simulink model "LICENTA_2024v8"  (R2018b)
settings: Solver=FixedStepDiscrete  StartTime=0.0  StopTime=Inf  RelTol=1e-3  EnableMultiTasking=on
values from neighbouring files (symbols this model uses):
  factor_conversie = (1/Rshunt)*(1/10)*(vref/4095)    (= 0.0115122972266)    [licentam18.m]
  FED = uint16(50)    [licentam18.m]
  MaxIter_1_ms_eCAP_wait = MinDetectSpeed_period/T_pos    (= 375)    [licentam18.m]
  offset_ADC = xT*4095/vref    (= 2047.5)    [licentam18.m]
  pp = 16/2    (= 8)    [licentam18.m]
  RED = uint16(50)    [licentam18.m]
  T_pos = 5*10^-4    (= 0.0005)    [licentam18.m]
  TBPRD1 = uint16(TPWM/(2*TTBCLK))    [licentam18.m]
  Tf = 0.015    [licentam18.m]
  Tf_spd = 0.01    [licentam18.m]
  TiSamplePos = T_pos    (= 0.0005)    [licentam18.m]
  Ts = Ts_crt_control    (= 3.33333333333e-05)    [licentam18.m]
  TTBCLK = 1/F    (= 5e-09)    [licentam18.m]
undefined symbols (not defined in the file or in its folder): Discrete, Down, GPTRIP1SEL, GPTRIP2SEL, radians, Time, TZ1, TZ2, Up
libraries: tiiqmathlib x25, c2802xlib x6, c2837xDlib x6, c280xlib x4, simulink x3, ctrlSharedLib x2, c2000lib x1, c28xdmclib x1
(part 2 of 2)

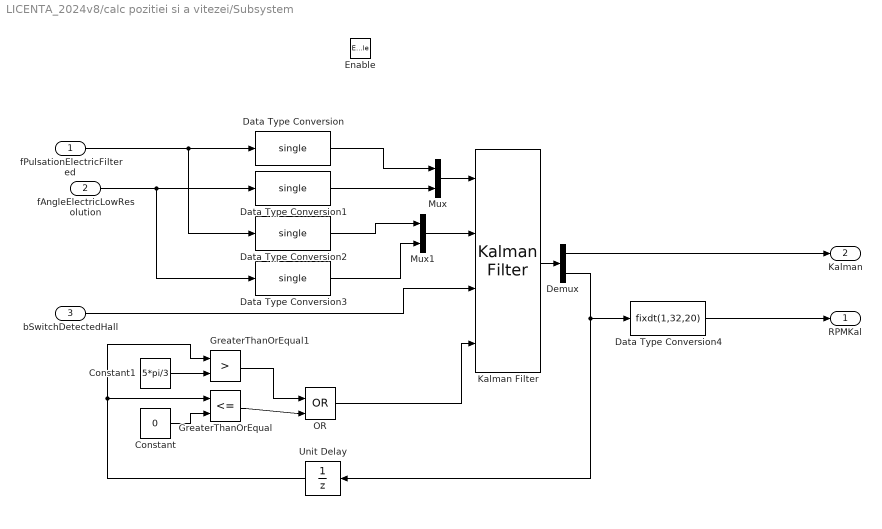
== system LICENTA_2024v8/calc pozitiei si a vitezei/Subsystem ==
  fPulsationElectricFiltered : Inport
  fAngleElectricLowResolution : Inport  Port=2
  bSwitchDetectedHall : Inport  Port=3
  Enable : EnablePort  StatesWhenEnabling=reset
  Constant : Constant  Value=0
  Constant1 : Constant  Value=5*pi/3
  Data Type Conversion{,1..3} (4 alike) : DataTypeConversion  OutDataTypeStr=single
  Data Type Conversion4 : DataTypeConversion  OutDataTypeStr=fixdt(1,32,20)
  Demux : Demux  Outputs=2
  GreaterThanOrEqual : RelationalOperator  Operator=<=  OutDataTypeStr=boolean  RndMeth=Simplest
  GreaterThanOrEqual1 : RelationalOperator  Operator=>  OutDataTypeStr=boolean  RndMeth=Simplest
  Kalman Filter : ctrlSharedLib/Kalman Filter  TimeDomain=Discrete-Time  UseCurrentEstimator=on  ModelSource=Individual A, B, C, D matrices  ModelSourceVariable=ss(0.95,1,1,0,1)  A=[1, 0; TiSamplePos 1]  B=1  C=eye(2)  D=0  NumberOfStates=1  NumberOfInputs=1  NumberOfOutputs=1  InitialEstimateSource=Input port  X0=0  P0=10  UseK=off  UseGH=off  NumberOfProcessNoiseInputs=1  G=1  TimeInvariantG=on  H=0  TimeInvariantH=on  Q=diag([0.00005 0.02])  TimeInvariantQ=on  R=diag([0.02 0.002])  TimeInvariantR=on  N=0  TimeInvariantN=on  AddInputPort=off  AddEnablePort=on  ExternalReset=Rising  OutputEstimatedY=off  OutputP=off  Ts=-1
      settings: SourceProductBaseCode=CT
  Mux : Mux  Inputs=2
  Mux1 : Mux  Inputs=2
  OR : Logic  Operator=OR  IconShape=distinctive  AllPortsSameDT=off  OutDataTypeStr=boolean
  Unit Delay : UnitDelay  SampleTime=-1
  RPMKal : Outport  VectorParamsAs1DForOutWhenUnconnected=on
  Kalman : Outport  Port=2
  wires:
  Kalman Filter/1 -> Demux/1
  Data Type Conversion3/1 -> Mux1/2
  Unit Delay/1 -> GreaterThanOrEqual/1, GreaterThanOrEqual1/1
  Data Type Conversion/1 -> Mux/1
  Constant/1 -> GreaterThanOrEqual/2
  Data Type Conversion1/1 -> Mux/2
  Data Type Conversion2/1 -> Mux1/1
  GreaterThanOrEqual/1 -> OR/2
  Constant1/1 -> GreaterThanOrEqual1/2
  Data Type Conversion4/1 -> RPMKal/1
  Mux/1 -> Kalman Filter/1
  Mux1/1 -> Kalman Filter/2
  OR/1 -> Kalman Filter/4
  GreaterThanOrEqual1/1 -> OR/1
  Demux/1 -> Kalman/1
  Demux/2 -> Unit Delay/1, Data Type Conversion4/1
  bSwitchDetectedHall/1 -> Kalman Filter/3
  fPulsationElectricFiltered/1 -> Data Type Conversion2/1, Data Type Conversion/1
  fAngleElectricLowResolution/1 -> Data Type Conversion3/1, Data Type Conversion1/1

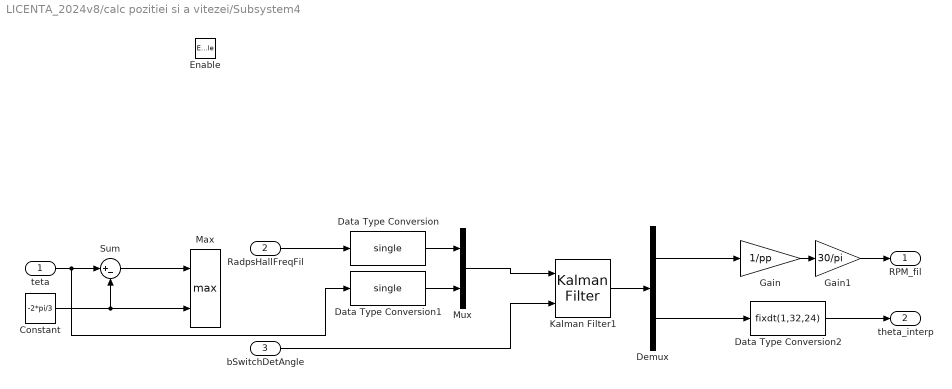
== system LICENTA_2024v8/calc pozitiei si a vitezei/Subsystem4 ==
  "teta " : Inport
  RadpsHallFreqFil : Inport  Port=2
  bSwitchDetAngle : Inport  Port=3
  Enable : EnablePort
  Constant : Constant  Value=-2*pi/3
  Data Type Conversion : DataTypeConversion  OutDataTypeStr=single
  Data Type Conversion1 : DataTypeConversion  OutDataTypeStr=single
  Data Type Conversion2 : DataTypeConversion  OutDataTypeStr=fixdt(1,32,24)
  Demux : Demux  Outputs=2
  Gain : Gain  Gain=1/pp
  Gain1 : Gain  Gain=30/pi
  Kalman Filter1 : ctrlSharedLib/Kalman Filter  TimeDomain=Discrete-Time  UseCurrentEstimator=on  ModelSource=Individual A, B, C, D matrices  ModelSourceVariable=sys  A=[1, 0; TiSamplePos 1]  B=eye(2)  C=eye(2)  D=zeros(2)  NumberOfStates=2  NumberOfInputs=2  NumberOfOutputs=2  InitialEstimateSource=Dialog  X0=0  P0=10  UseK=off  UseGH=off  NumberOfProcessNoiseInputs=2  G=1  TimeInvariantG=on  H=0  TimeInvariantH=on  Q=diag([0.2 0.5])  TimeInvariantQ=on  R=diag([2.5 0.001])  TimeInvariantR=on  N=0  TimeInvariantN=on  AddInputPort=off  AddEnablePort=on  OutputEstimatedY=off  OutputP=off  Ts=-1
      settings: SourceProductBaseCode=CT
  Max : MinMax  Function=max  Inputs=2
  Mux : Mux  Inputs=2
  Sum : Sum  Inputs=|+-
  RPM_fil : Outport
  theta_interp : Outport  Port=2
  wires:
  Data Type Conversion2/1 -> theta_interp/1
  Gain1/1 -> RPM_fil/1
  Demux/2 -> Data Type Conversion2/1
  Gain/1 -> Gain1/1
  Demux/1 -> Gain/1
  Kalman Filter1/1 -> Demux/1
  bSwitchDetAngle/1 -> Kalman Filter1/2
  Mux/1 -> Kalman Filter1/1
  Data Type Conversion1/1 -> Mux/2
  Data Type Conversion/1 -> Mux/1
  RadpsHallFreqFil/1 -> Data Type Conversion/1
  Sum/1 -> Max/1
  Constant/1 -> Max/2, Sum/2
  "teta "/1 -> Data Type Conversion1/1, Sum/1

== system LICENTA_2024v8/calc pozitiei si a vitezei/calc pozitie ==
  In1 : Inport
  Data Type Conversion : DataTypeConversion  OutDataTypeStr=int8
  MATLAB Function : MATLAB Function  TreatAsAtomicUnit=on
  citire senzori hall & calcul teta : Subsystem
  gradient : Subsystem
  teta : Outport  VectorParamsAs1DForOutWhenUnconnected=on
  int8dir : Outport  Port=2  VectorParamsAs1DForOutWhenUnconnected=on
  "seq. change detected " : Outport  Port=3  VectorParamsAs1DForOutWhenUnconnected=on
  wires:
  Data Type Conversion/1 -> int8dir/1
  MATLAB Function/1(dir) -> Data Type Conversion/1
  gradient/1(gradient) -> MATLAB Function/1(u)
  citire senzori hall & calcul teta/1(teta) -> teta/1, gradient/1(teta)
  citire senzori hall & calcul teta/2("seq. change detected ") -> "seq. change detected "/1, gradient/Trigger
  In1/1 -> citire senzori hall & calcul teta/1(In1)

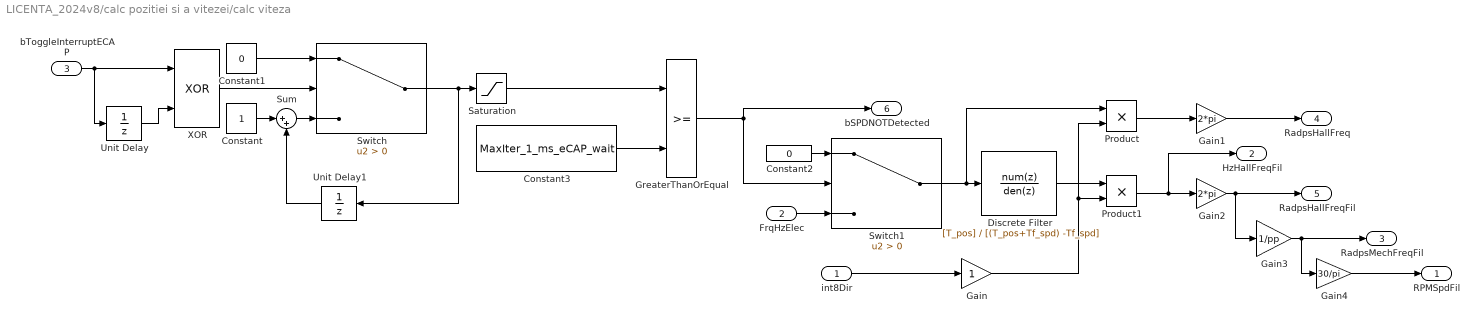
== system LICENTA_2024v8/calc pozitiei si a vitezei/calc viteza ==
  int8Dir : Inport
  FrqHzElec : Inport  Port=2
  bToggleInterruptECAP : Inport  Port=3
  Constant : Constant
  Constant1 : Constant  Value=0
  Constant2 : Constant  Value=0
  Constant3 : Constant  Value=MaxIter_1_ms_eCAP_wait
  Discrete Filter : DiscreteFilter  Numerator=[T_pos]  Denominator=[(T_pos+Tf_spd) -Tf_spd]
  Gain : Gain
  Gain1 : Gain  Gain=2*pi
  Gain2 : Gain  Gain=2*pi
  Gain3 : Gain  Gain=1/pp
  Gain4 : Gain  Gain=30/pi
  GreaterThanOrEqual : RelationalOperator  OutDataTypeStr=boolean  RndMeth=Simplest
  Product : Product
  Product1 : Product
  Saturation : Saturate  UpperLimit=MaxIter_1_ms_eCAP_wait  LowerLimit=0
  Sum : Sum  Inputs=|++
  Switch : Switch  Criteria=u2 > Threshold
  Switch1 : Switch  Criteria=u2 > Threshold
  Unit Delay : UnitDelay  SampleTime=-1
  Unit Delay1 : UnitDelay  SampleTime=-1
  XOR : Logic  Operator=XOR  IconShape=distinctive  AllPortsSameDT=off  OutDataTypeStr=boolean
  RPMSpdFil : Outport  VectorParamsAs1DForOutWhenUnconnected=on
  HzHallFreqFil : Outport  Port=2  VectorParamsAs1DForOutWhenUnconnected=on
  RadpsMechFreqFil : Outport  Port=3  VectorParamsAs1DForOutWhenUnconnected=on
  RadpsHallFreq : Outport  Port=4  VectorParamsAs1DForOutWhenUnconnected=on
  RadpsHallFreqFil : Outport  Port=5  VectorParamsAs1DForOutWhenUnconnected=on
  bSPDNOTDetected : Outport  Port=6  VectorParamsAs1DForOutWhenUnconnected=on
  wires:
  Constant2/1 -> Switch1/1
  FrqHzElec/1 -> Switch1/3
  Sum/1 -> Switch/3
  Unit Delay/1 -> XOR/2
  Saturation/1 -> GreaterThanOrEqual/1
  bToggleInterruptECAP/1 -> XOR/1, Unit Delay/1
  Unit Delay1/1 -> Sum/2
  Switch/1 -> Unit Delay1/1, Saturation/1
  Constant/1 -> Sum/1
  Product1/1 -> Gain2/1, HzHallFreqFil/1
  XOR/1 -> Switch/2
  Product/1 -> Gain1/1
  Constant3/1 -> GreaterThanOrEqual/2
  Gain1/1 -> RadpsHallFreq/1
  Gain/1 -> Product1/2, Product/2
  Constant1/1 -> Switch/1
  Gain4/1 -> RPMSpdFil/1
  Gain2/1 -> Gain3/1, RadpsHallFreqFil/1
  GreaterThanOrEqual/1 -> Switch1/2, bSPDNOTDetected/1
  Gain3/1 -> Gain4/1, RadpsMechFreqFil/1
  Discrete Filter/1 -> Product1/1
  int8Dir/1 -> Gain/1
  Switch1/1 -> Product/1, Discrete Filter/1

== system LICENTA_2024v8/eCAP/If Action Subsystem ==
  HzHallFreqPrev : Inport
  Action Port : ActionPort  ActionType=then
  HzHallFreq : Outport  VectorParamsAs1DForOutWhenUnconnected=on
  wires:
  HzHallFreqPrev/1 -> HzHallFreq/1

== system LICENTA_2024v8/eCAP/If Action Subsystem1 ==
  Action Port : ActionPort  ActionType=elseif
  Constant : Constant  Value=0
  HzHallFreq : Outport  VectorParamsAs1DForOutWhenUnconnected=on
  wires:
  Constant/1 -> HzHallFreq/1

== system LICENTA_2024v8/eCAP/If Action Subsystem2 ==
  HallPeriod : Inport
  Action Port : ActionPort  ActionType=else
  Constant : Constant
  Multiply : Product  Inputs=*/
  HzHallFreq : Outport  VectorParamsAs1DForOutWhenUnconnected=on
  wires:
  HallPeriod/1 -> Multiply/2
  Constant/1 -> Multiply/1
  Multiply/1 -> HzHallFreq/1

== system LICENTA_2024v8/calc pozitiei si a vitezei/calc pozitie/citire senzori hall & calcul teta ==
  In1 : Inport
  Digital Input : c2837xDlib/Digital Input  GPIO_Number=GPIO24~GPIO31  GPIO_Bit0=off  GPIO_Bit1=off  GPIO_Bit2=on  GPIO_Bit3=off  GPIO_Bit4=off  GPIO_Bit5=off  GPIO_Bit6=off  GPIO_Bit7=off  sampleTime=-1  dataType=auto  GPIO_Bit0_Qualification=Sync to SYSCLKOUT  GPIO_Bit1_Qualification=Sync to SYSCLKOUT  GPIO_Bit2_Qualification=Sync to SYSCLKOUT  GPIO_Bit3_Qualification=Sync to SYSCLKOUT  GPIO_Bit4_Qualification=Sync to SYSCLKOUT  GPIO_Bit5_Qualification=Sync to SYSCLKOUT  GPIO_Bit6_Qualification=Sync to SYSCLKOUT  GPIO_Bit7_Qualification=Sync to SYSCLKOUT  Qualification_Period=-1
      settings: SourceProductBaseCode=TIC2000
  Digital Input1 : c2837xDlib/Digital Input  GPIO_Number=GPIO24~GPIO31  GPIO_Bit0=off  GPIO_Bit1=off  GPIO_Bit2=off  GPIO_Bit3=on  GPIO_Bit4=off  GPIO_Bit5=off  GPIO_Bit6=off  GPIO_Bit7=off  sampleTime=-1  dataType=auto  GPIO_Bit0_Qualification=Sync to SYSCLKOUT  GPIO_Bit1_Qualification=Sync to SYSCLKOUT  GPIO_Bit2_Qualification=Sync to SYSCLKOUT  GPIO_Bit3_Qualification=Sync to SYSCLKOUT  GPIO_Bit4_Qualification=Sync to SYSCLKOUT  GPIO_Bit5_Qualification=Sync to SYSCLKOUT  GPIO_Bit6_Qualification=Sync to SYSCLKOUT  GPIO_Bit7_Qualification=Sync to SYSCLKOUT  Qualification_Period=-1
      settings: SourceProductBaseCode=TIC2000
  Digital Input2 : c2837xDlib/Digital Input  GPIO_Number=GPIO24~GPIO31  GPIO_Bit0=off  GPIO_Bit1=on  GPIO_Bit2=off  GPIO_Bit3=off  GPIO_Bit4=off  GPIO_Bit5=off  GPIO_Bit6=off  GPIO_Bit7=off  sampleTime=-1  dataType=auto  GPIO_Bit0_Qualification=Sync to SYSCLKOUT  GPIO_Bit1_Qualification=Sync to SYSCLKOUT  GPIO_Bit2_Qualification=Sync to SYSCLKOUT  GPIO_Bit3_Qualification=Sync to SYSCLKOUT  GPIO_Bit4_Qualification=Sync to SYSCLKOUT  GPIO_Bit5_Qualification=Sync to SYSCLKOUT  GPIO_Bit6_Qualification=Sync to SYSCLKOUT  GPIO_Bit7_Qualification=Sync to SYSCLKOUT  Qualification_Period=-1
      settings: SourceProductBaseCode=TIC2000
  Optimizare : Subsystem
  transf clarke : Subsystem
  teta : Outport  VectorParamsAs1DForOutWhenUnconnected=on
  "seq. change detected " : Outport  Port=2
  wires:
  Digital Input2/1 -> transf clarke/1(HallA), Optimizare/1(HallA)
  Digital Input/1 -> transf clarke/2(HallB), Optimizare/2(HallB)
  Digital Input1/1 -> transf clarke/3(HallC), Optimizare/3(HallC)
  Optimizare/1("seq. change detected ") -> "seq. change detected "/1, transf clarke/Trigger
  transf clarke/1(teta) -> teta/1
  In1/1 -> transf clarke/4(teta_allighn)

== system LICENTA_2024v8/calc pozitiei si a vitezei/calc pozitie/gradient ==
  teta : Inport
  Trigger : TriggerPort  VariantControl=Variant  PortDimensions=1
  Sum : Sum  Inputs=+-
  Unit Delay : UnitDelay  SampleTime=-1
  gradient : Outport  VectorParamsAs1DForOutWhenUnconnected=on
  wires:
  Unit Delay/1 -> Sum/2
  Sum/1 -> gradient/1
  teta/1 -> Sum/1, Unit Delay/1

== system LICENTA_2024v8/calc pozitiei si a vitezei/calc pozitie/citire senzori hall & calcul teta/Optimizare ==
  HallA : Inport
  HallB : Inport  Port=2
  HallC : Inport  Port=3
  Unit Delay : UnitDelay  SampleTime=-1
  Unit Delay1 : UnitDelay  SampleTime=-1
  Unit Delay2 : UnitDelay  SampleTime=-1
  XOR : Logic  Operator=XOR  Inputs=6  AllPortsSameDT=off  OutDataTypeStr=boolean
  "seq. change detected " : Outport  VectorParamsAs1DForOutWhenUnconnected=on
  wires:
  XOR/1 -> "seq. change detected "/1
  Unit Delay1/1 -> XOR/6
  Unit Delay2/1 -> XOR/5
  HallC/1 -> XOR/3, Unit Delay1/1
  HallA/1 -> XOR/1, Unit Delay/1
  Unit Delay/1 -> XOR/4
  HallB/1 -> XOR/2, Unit Delay2/1

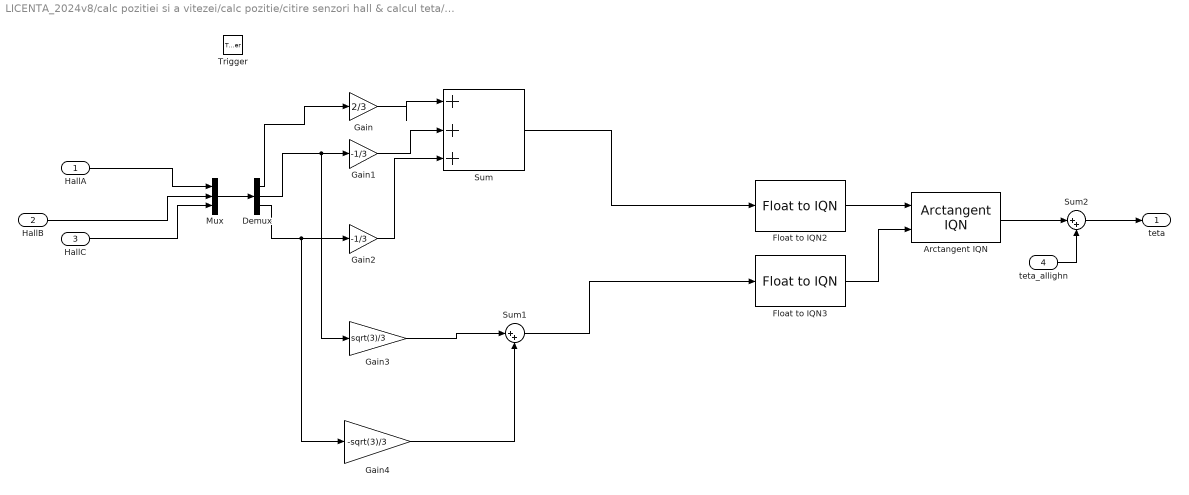
== system LICENTA_2024v8/calc pozitiei si a vitezei/calc pozitie/citire senzori hall & calcul teta/transf clarke ==
  HallA : Inport
  HallB : Inport  Port=2
  HallC : Inport  Port=3
  teta_allighn : Inport  Port=4
  Trigger : TriggerPort  VariantControl=(inherit)  PortDimensions=1
  Arctangent IQN : tiiqmathlib/Arctangent IQN  tanOption=atan2 (radians)
      settings: SourceProductBaseCode=TIC2000
  Demux : Demux  Outputs=3
  Float to IQN2 : tiiqmathlib/Float to IQN  Q_value=20
      settings: SourceProductBaseCode=TIC2000
  Float to IQN3 : tiiqmathlib/Float to IQN  Q_value=20
      settings: SourceProductBaseCode=TIC2000
  Gain : Gain  Gain=2/3
  Gain1 : Gain  Gain=-1/3
  Gain2 : Gain  Gain=-1/3
  Gain3 : Gain  Gain=sqrt(3)/3
  Gain4 : Gain  Gain=-sqrt(3)/3
  Mux : Mux  Inputs=3
  Sum : Sum  Inputs=|+++  OutDataTypeStr=single
  Sum1 : Sum  Inputs=|++  AccumDataTypeStr=single
  Sum2 : Sum  Inputs=|++
  teta : Outport  VectorParamsAs1DForOutWhenUnconnected=on
  wires:
  Mux/1 -> Demux/1
  HallC/1 -> Mux/3
  HallB/1 -> Mux/2
  HallA/1 -> Mux/1
  Gain3/1 -> Sum1/1
  Gain4/1 -> Sum1/2
  Gain2/1 -> Sum/3
  Gain1/1 -> Sum/2
  Demux/3 -> Gain2/1, Gain4/1
  Gain/1 -> Sum/1
  Demux/2 -> Gain1/1, Gain3/1
  Demux/1 -> Gain/1
  Float to IQN2/1 -> Arctangent IQN/1
  Float to IQN3/1 -> Arctangent IQN/2
  Sum1/1 -> Float to IQN3/1
  Sum/1 -> Float to IQN2/1
  Sum2/1 -> teta/1
  teta_allighn/1 -> Sum2/2
  Arctangent IQN/1 -> Sum2/1

== matlab function LICENTA_2024v8/calc pozitiei si a vitezei/calc pozitie/MATLAB Function ==
  data: u input; dir output
function dir = fcn(u)

persistent dir_prev;
if isempty(dir_prev)
    dir_prev=0;
end
if (u < -2 || u > 2)
    dir=dir_prev;
else
    if u > 0.5
        dir = 1;
    elseif u < -0.5
        dir = -1;
    else
        dir = 0;
    end
end
dir_prev=dir;
